simulink model "task_1_lin"  (R2024a)
settings: Solver=VariableStepAuto  StartTime=0.0  StopTime=75  MaxStep=1e-4  RelTol=1e-4
values from neighbouring files (symbols this model uses):
  f = Y_f * w    [pendulum_ode_with_compensation.m]
undefined symbols (not defined in the file or in its folder): A, B, C, D, K, x_0
settings Model: Creator=user  LastModifiedBy=user
settings RTWCC: GPUComputeCapability=3.5

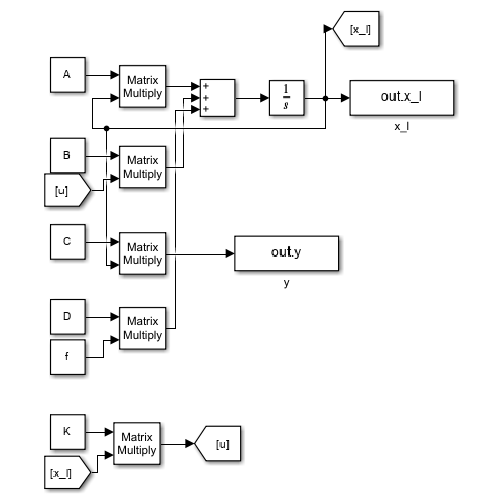
[thumbnail: Simulink's stored preview of the top-level diagram]
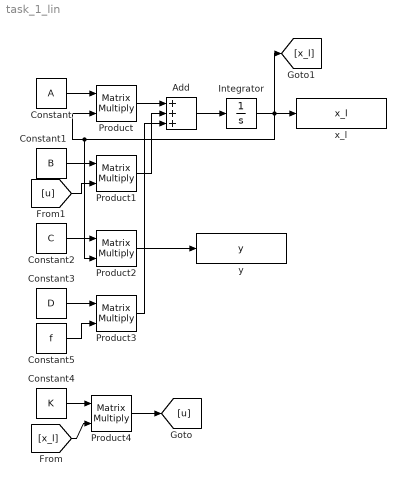
== system task_1_lin ==
  Add : Sum  Inputs=+++
  Constant : Constant  Value=A  VectorParams1D=off
  Constant1 : Constant  Value=B  VectorParams1D=off
  Constant2 : Constant  Value=C  VectorParams1D=off
  Constant3 : Constant  Value=D  VectorParams1D=off
  Constant4 : Constant  Value=K  VectorParams1D=off
  Constant5 : Constant  Value=f  VectorParams1D=off
  Integrator : Integrator  InitialCondition=x_0
  Product{,1..4} (5 alike) : Product  Multiplication=Matrix(*)
  x_l : ToWorkspace  VariableName=x_l  SaveFormat=Timeseries  SampleTime=-1
  y : ToWorkspace  VariableName=y  SaveFormat=Timeseries  SampleTime=-1
  wires:
  Constant/1 -> Product/1
  Constant1/1 -> Product1/1
  Integrator/1 -> [x_l], Product2/2, Product/2, x_l/1
  Constant2/1 -> Product2/1
  Product2/1 -> y/1
  Constant3/1 -> Product3/1
  Constant5/1 -> Product3/2
  Add/1 -> Integrator/1
  Product/1 -> Add/1
  Product1/1 -> Add/2
  Product3/1 -> Add/3
  Constant4/1 -> Product4/1
  [x_l] -> Product4/2
  Product4/1 -> [u]
  [u] -> Product1/2
